simulink model "Decode_Encode_Num"  (R2017a)
settings: Solver=VariableStepAuto  StartTime=0.0  StopTime=1  RelTol=1e-3
settings Model: Creator=telep  LastModifiedBy=telep

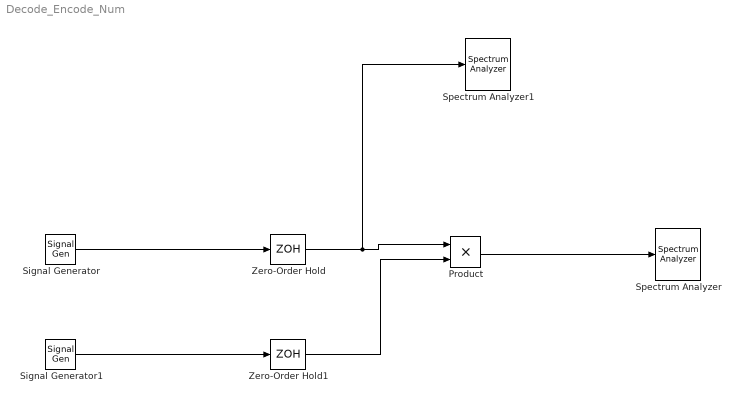
== system Decode_Encode_Num ==
  Product : Product
  Signal Generator : SignalGenerator  WaveForm=square  Frequency=1/0.002
  Signal Generator1 : SignalGenerator  WaveForm=square  Frequency=28000
  Spectrum Analyzer : SpectrumAnalyzer
  Spectrum Analyzer1 : SpectrumAnalyzer
  Zero-Order Hold : ZeroOrderHold  SampleTime=1/28000
  Zero-Order Hold1 : ZeroOrderHold  SampleTime=1/28000
  wires:
  Signal Generator/1 -> Zero-Order Hold/1
  Signal Generator1/1 -> Zero-Order Hold1/1
  Zero-Order Hold/1 -> Spectrum Analyzer1/1, Product/1
  Zero-Order Hold1/1 -> Product/2
  Product/1 -> Spectrum Analyzer/1
